simulink model "twelvepulserectkir"  (R2023a)
settings: Solver=ode45  StartTime=0.0  StopTime=1.0  RelTol=1e-3
undefined symbols (not defined in the file): D11, Delta
libraries: spsDiodeLib x12, spsACVoltageSourceLib x3, spsCurrentMeasurementLib x3, spsGroundLib x1, spsSeriesRLCBranchLib x1, spsThreePhaseTransformerThreeWindingsLib x1, spsVoltageMeasurementLib x1, sps_lib x1
settings Model: Creator=Kiran D Gowda  LastModifiedBy=Kiran D Gowda

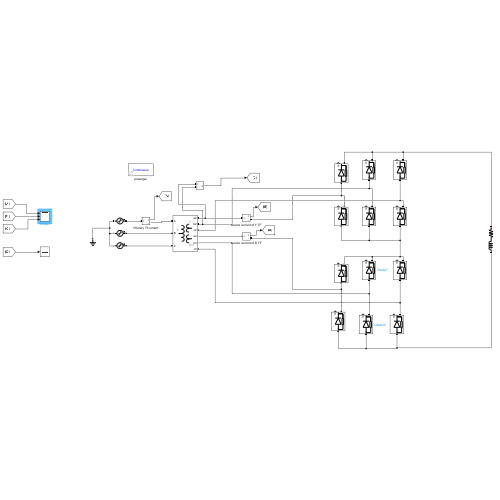
[thumbnail: Simulink's stored preview of the top-level diagram]
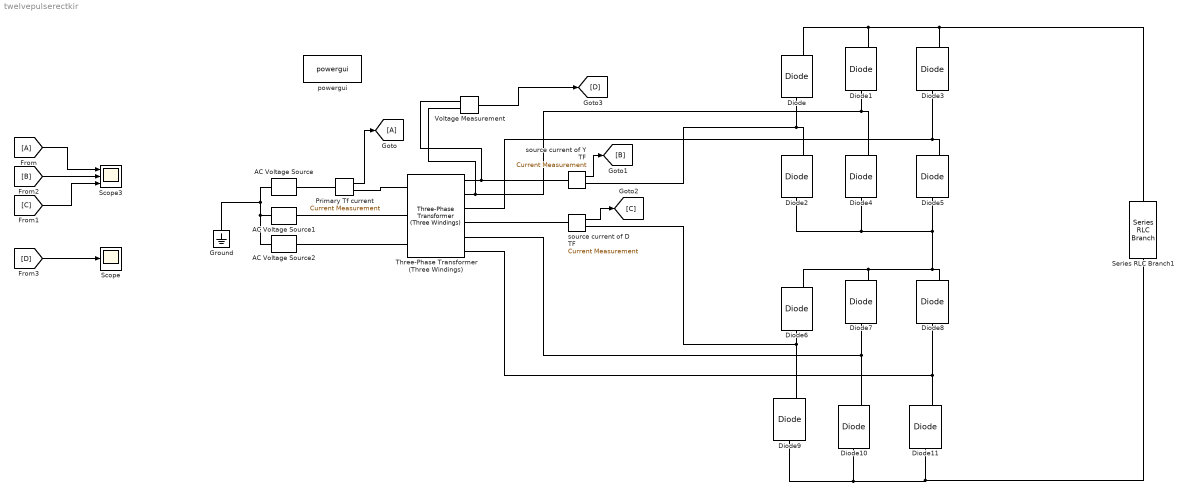
== system twelvepulserectkir ==
  AC Voltage Source : spsACVoltageSourceLib/AC Voltage Source  Amplitude=100  Phase=0  Frequency=50  SampleTime=0  Measurements=Voltage  BusType=swing  Pref=10e3  Qref=0  Qmin=-inf  Qmax=+inf
  AC Voltage Source1 : spsACVoltageSourceLib/AC Voltage Source  Amplitude=100  Phase=-120  Frequency=50  SampleTime=0  Measurements=Voltage  BusType=swing  Pref=10e3  Qref=0  Qmin=-inf  Qmax=+inf
  AC Voltage Source2 : spsACVoltageSourceLib/AC Voltage Source  Amplitude=100  Phase=-240  Frequency=50  SampleTime=0  Measurements=Voltage  BusType=swing  Pref=10e3  Qref=0  Qmin=-inf  Qmax=+inf
  Diode{,1..11} (12 alike) : spsDiodeLib/Diode  Ron=0.001  Lon=0  Vf=0.8  IC=0  UseSnubber=0  Rs=500  Cs=250e-9  Measurements=on
  From : From
  Goto : Goto
  Ground : spsGroundLib/Ground  LConnTagsString=a
  Primary Tf current : spsCurrentMeasurementLib/Current Measurement  PhasorSimulation=off  OutputType=Complex  PSBequivalent=0
  Scope : Scope
  Scope3 : Scope  NumInputPorts=3
  Series RLC Branch1 : spsSeriesRLCBranchLib/Series RLC Branch  LConnTagsString=__new0  RConnTagsString=__new0  BranchType=RL  Resistance=500  Inductance=500e-3  SetiL0=off  InitialCurrent=0  Capacitance=1e-6  Setx0=off  InitialVoltage=0  Measurements=Branch voltage and current
  Three-Phase Transformer (Three Windings) : spsThreePhaseTransformerThreeWindingsLib/Three-Phase Transformer (Three Windings)  Winding1Connection=Y  Winding2Connection=Y  Winding3Connection=Delta (D11)  CoreType=Three-limb core (core-type)  SetSaturation=off  Hysteresis=off  DataFile='hysteresis'  SetInitialFlux=off  Measurements=All measurements (V I Fluxes)  UNITS=SI  NominalPower=[ 250e6 , 50 ]  Winding1=[100 0 0.015]  Winding2=[50 0 0.015]  Winding3=[50 0 0.015]  Rm=10000  Lm=2866  L0=1000  Saturation=[0 0;0.66653 1910.3;277.72 2419.7]  InitialFluxes=[0.8 -0.8 0.7]  BreakLoop=off  DiscreteSolver=Trapezoidal iterative  DataType=on  TransfoNumber=1
      settings: LibrarySourceBlock=|
      | sps_lib/Power Grid Elements/Three-Phase
      | Transformer
      | (Three Windings)
  Voltage Measurement : spsVoltageMeasurementLib/Voltage Measurement  PhasorSimulation=off  OutputType=Complex  PSBequivalent=0
  powergui : sps_lib/powergui  Priority=1  SimulationMode=Continuous  SampleTime=1e-6  frequency=60  Iterations=50  frequencyindice=50  Pbase=100e6  ErrMax=1e-4  UnitsV=kV  UnitsW=MW  buscounter=0  FunctionMessages=off  echomessages=off  EnableUseOfTLC=off  CurrentSourceSwitches=off  DisableSnubberDevices=off  DisableRonSwitches=off  DisableVfSwitches=off  DisplayEquations=off  AutomaticDiscreteSolvers=off  SolverType=Tustin/Backward Euler (TBE)  Interpol=off  ExternalGateDelay=off  methode=off  Ts=100  x0status=blocks  SPID=on  SwTol=0  HookPort=off  NonlinearTolerance=1e-4  nMaxIteration=100  ContinueOnMaxIteration=off  RestoreLinks=warning  ResistiveCurrentMeasurement=off  Frange=[0:2:500]  Ylog=off  Xlog=on  ShowGrid=off  save=off  variable=ZData  structure=0  ZoomFFT=off  StartTime=0.0  cycles=1  DisplayStyle=1  fundamental=60  FreqAxis=off  MaxFrequency=1000  frequencyindicesteady=1  RmsSteady=1  display=off
  source current of D TF : spsCurrentMeasurementLib/Current Measurement  PhasorSimulation=off  OutputType=Complex  PSBequivalent=0
  source current of Y TF : spsCurrentMeasurementLib/Current Measurement  PhasorSimulation=off  OutputType=Complex  PSBequivalent=0
  wires:
  Primary Tf current/1 -> Goto/1
  source current of Y TF/1 -> [B]
  source current of D TF/1 -> [C]
  From/1 -> Scope3/1
  [C] -> Scope3/3
  [B] -> Scope3/2
  Voltage Measurement/1 -> [D]
  [D] -> Scope/1
  connections:
  AC Voltage Source1/LConn1 -- AC Voltage Source2/LConn1 -- AC Voltage Source/LConn1 -- Ground/LConn1
  AC Voltage Source2/RConn1 -- Three-Phase Transformer (Three Windings)/LConn3
  AC Voltage Source1/RConn1 -- Three-Phase Transformer (Three Windings)/LConn2
  source current of Y TF/RConn1 -- Diode2/RConn1 -- Diode/LConn1
  Voltage Measurement/LConn2 -- Three-Phase Transformer (Three Windings)/RConn2 -- Diode4/RConn1 -- Diode1/LConn1
  Three-Phase Transformer (Three Windings)/RConn3 -- Diode5/RConn1 -- Diode3/LConn1
  Series RLC Branch1/LConn1 -- Diode3/RConn1 -- Diode1/RConn1 -- Diode/RConn1
  Three-Phase Transformer (Three Windings)/RConn5 -- Diode7/LConn1 -- Diode10/RConn1
  Three-Phase Transformer (Three Windings)/RConn6 -- Diode8/LConn1 -- Diode11/RConn1
  source current of D TF/RConn1 -- Diode9/RConn1 -- Diode6/LConn1
  Three-Phase Transformer (Three Windings)/RConn1 -- Voltage Measurement/LConn1 -- source current of Y TF/LConn1
  Three-Phase Transformer (Three Windings)/RConn4 -- source current of D TF/LConn1
  AC Voltage Source/RConn1 -- Primary Tf current/LConn1
  Primary Tf current/RConn1 -- Three-Phase Transformer (Three Windings)/LConn1
  Diode11/LConn1 -- Series RLC Branch1/RConn1 -- Diode10/LConn1 -- Diode9/LConn1
  Diode2/LConn1 -- Diode7/RConn1 -- Diode6/RConn1 -- Diode8/RConn1 -- Diode5/LConn1 -- Diode4/LConn1
